simulink model "Ej2L"  (Simulink 8.3)
settings: Solver=ode45  StartTime=0.0  StopTime=10.0  RelTol=1e-3
settings Model: Creator=gasti  LastModifiedBy=gasti
settings DataIOCC: SignalLoggingSaveFormat=Dataset
settings DebuggingCC: UnderspecifiedInitializationDetection=Simplified  StateNameClashWarn=none
settings GRTTargetCC: CombineOutputUpdateFcns=on  GRTInterface=off

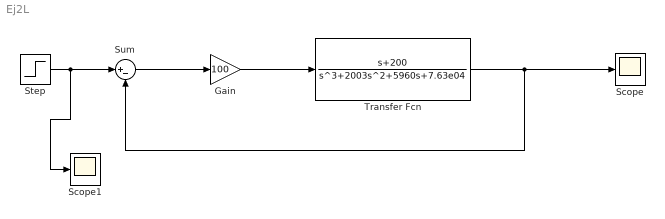
== system Ej2L ==
  Gain : Gain  Gain=100
  Scope : Scope
  Scope1 : Scope
  Step : Step  Before=2  After=5  SampleTime=0
  Sum : Sum  Inputs=|+-
  Transfer Fcn : TransferFcn  Numerator=[1 200]  Denominator=[1 2003 5960 7.63e04]
  wires:
  Gain/1 -> Transfer Fcn/1
  Transfer Fcn/1 -> Scope/1, Sum/2
  Sum/1 -> Gain/1
  Step/1 -> Scope1/1, Sum/1
